simulink model "Controller_Sim"  (R2016a)
settings: Solver=ode1  SolverMode=MultiTasking  StartTime=0.0  StopTime=10  FixedStep=0.0005  RelTol=1e-3
StopFcn:
  | structifySimData
  | ConstructLog_Sim
values from neighbouring files (symbols this model uses):
  ControlParams = input.ControlParams    [Controller.m]    (also in Controller_Yukai.m)
  ControlState = input.ControlState    [Controller.m]    (also in Controller_Yukai.m)
undefined symbols (not defined in the file or in its folder): DiscIntNeverNeededParam, EnablePerturb, EnableStictionModel, FootPoints, gd, get, GroundModel, leg_length, LegHipTorqueLimit, LibWalkingDDA, pL1, pL2, pR1, pR2, ps3Axes, ps3Buttons, ps3Pov, RoughTerrain1, spring_k, spring_zeta, torso_com_offset, Ts, xinit, xLine, yLine, Z
libraries: simulink x5, Friction_Compensator_Lib x2, robotlib x2, vrlib x1
(part 1 of 2)
settings Model: ParamWorkspaceSource=ReferencedWorkspace  TunableVars=AllowDoubleSupport,Alpha0Frottement,Alpha2Frottement,BoomParams,ControlParams,ControlState,ControllerModeInit,EnablePerturb,EnableTransition,EnergyControlGain,EnergyControlPhi0,GaitLibrary,HipPushMag,KASaturationEarly,KASaturationMax,KASaturationS1,KASaturationS2,KASpringOffsets,KContact,KZeroYaw,K_sha,K_sla,Ksqrt,KsqrtVert,LambdaContact,LegHipTorqueLimit,MinDeltaThetaTransition,ProjectTo2D,RunMode,SWAP_DELAY,StanceLegInit,TMaxUpdate,TPosing,TorsoBackAngle,TorsoBackOnStep,TransitionOutputParams,UseKASaturation,UsePosingControl,VBLAOptions,WalkingOutputParams,balanceParams,enable_dx_tgt,enable_dy_tgt,enable_sideStep,enable_yawControl,epsilon,ff_params,foot_adjust_params,foot_geometry,foot_points,ground_coefficient_of_friction,ground_height_data,h_alpha_nom,h_alpha_transition,hd_posing,isTest_constantHips,isTest_doubleSupport,isTest_hipTracking,isTest_holdInAir,isTest_stopAndGo,k_precomp,kd,kd_2dof,kd_hip,kd_pitch,kd_roll,kd_sha,kd_sla,kd_st_leg,kd_stanceHip,kd_stanceKnee,kd_stanceLeg,kd_sw_leg,kd_swingHip,kd_swingKnee,kd_swingLeg,kd_torso,ki_sha,ki_sla,kp,kp_2dof,kp_hip,kp_pitch,kp_roll,kp_sha,kp_sla,kp_st_leg,kp_stanceHip,kp_stanceKnee,kp_stanceLeg,kp_sw_leg,kp_swingHip,kp_swingKnee,kp_swingLeg,kp_torso,kp_yaw,lat_bias,lateralParams,optimal_sat_weights,pBInitial,ps3Axes,ps3Buttons,ps3Pov,springDeflectionImpactThreshold,spring_k,spring_zeta,stepTime,step_params,swap_params,swingHipAdjustmentGain,swingLegAdjustmentGain,tStepInitial,theta_limits_nom,theta_limits_transition,thres_hi,thres_lo,transitionParams,uHipGravity,u_ff,use2DOFHipControl,useConstantDecoupling,useOptimalSaturation,use_state_estimator,viscous_friction_yaw_constant,w_torso_lat,xinit  TunableVarsStorageClass=Auto,Auto,Auto,Auto,Auto,Auto,Auto,Auto,Auto,Auto,Auto,Auto,Auto,Auto,Auto,Auto,Auto,Auto,Auto,Auto,Auto,Auto,Auto,Auto,Auto,Auto,Auto,Auto,Auto,Auto,Auto,Auto,Auto,Auto,Auto,Auto,Auto,Auto,Auto,Auto,Auto,Auto,Auto,Auto,Auto,Auto,Auto,Auto,Auto,Auto,Auto,Auto,Auto,Auto,Auto,Auto,Auto,Auto,Auto,Auto,Auto,Auto,Auto,Auto,Auto,Auto,Auto,Auto,Auto,Auto,Auto,Auto,Auto,Auto,Auto,Auto,Auto,Auto,Auto,Auto,Auto,Auto,Auto,Auto,Auto,Auto,Auto,Auto,Auto,Auto,Auto,Auto,Auto,Auto,Auto,Auto,Auto,Auto,Auto,Auto,Auto,Auto,Auto,Auto,Auto,Auto,Auto,Auto,Auto,Auto,Auto,Auto,Auto,Auto,Auto,Auto,Auto,Auto,Auto,Auto,Auto,Auto,Auto,Auto,Auto,Auto  TunableVarsTypeQualifier=,,,,,,,,,,,,,,,,,,,,,,,,,,,,,,,,,,,,,,,,,,,,,,,,,,,,,,,,,,,,,,,,,,,,,,,,,,,,,,,,,,,,,,,,,,,,,,,,,,,,,,,,,,,,,,,,,,,,,,,,,,,,,  Creator=kevinsg  LastModifiedBy=gyk
settings SolverCC: AlgebraicLoopSolver=LineSearch
settings DataIOCC: LimitDataPoints=on  SaveFormat=Array
settings OptimizationCC: BlockReduction=off  BooleanDataType=off
settings DebuggingCC: SaveWithParameterizedLinksMsg=none  SignalResolutionControl=TryResolveAllWithWarning  AllowSymbolicDim=off
settings HardwareCC: ProdBitPerPointer=32  ProdLargestAtomicFloat=None  ProdIntDivRoundTo=Undefined  ProdEndianess=Unspecified  ProdWordSize=32  ProdHWDeviceType=32-bit Generic  TargetBitPerPointer=64  TargetLongLongMode=on  TargetIntDivRoundTo=Zero  TargetEndianess=LittleEndian  TargetWordSize=64  TargetHWDeviceType=MATLAB Host  ProdEqTarget=off
settings ModelReferenceCC: PropagateSignalLabelsOutOfModel=off
settings ConfigComp: CovModelRefEnable=Off  CovSFcnEnable=off

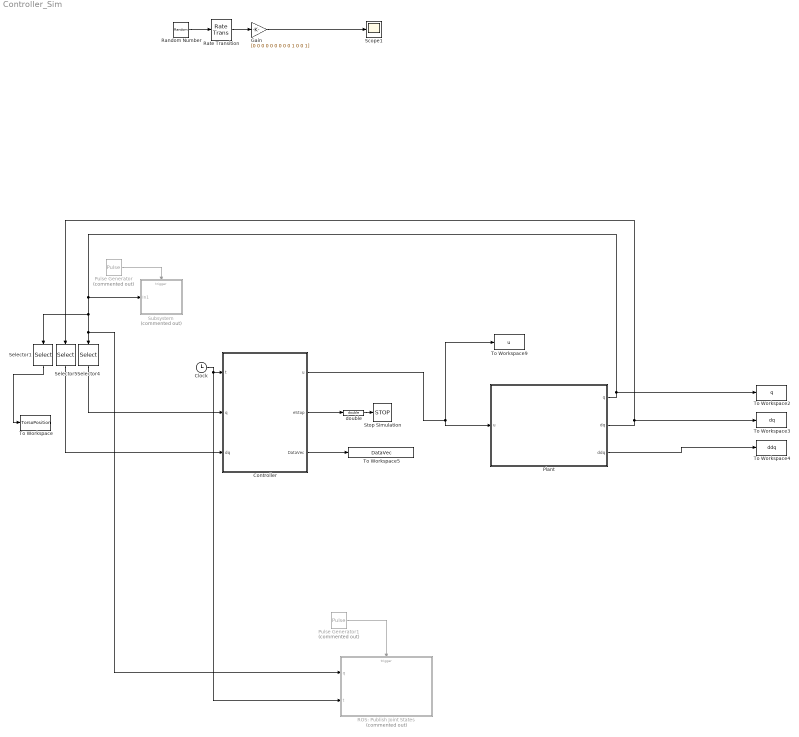
== system Controller_Sim ==
  Clock : Clock
  Controller : Subsystem  AncestorBlock=LibWalkingDDA/RoughTerrain1
  Gain : Gain  Gain=[0 0 0 0 0 0 0 0 0 1 0 0 1]
  Plant : Subsystem
  Pulse Generator : DiscretePulseGenerator  Commented=on  PulseType=Time based  Period=.01  PulseWidth=5
  Pulse Generator1 : DiscretePulseGenerator  Commented=on  PulseType=Time based  Period=.01  PulseWidth=5
  ROS: Publish Joint States : Subsystem  Commented=on
  Random Number : RandomNumber  Variance=Ts*300  SampleTime=Ts*100
  Rate Transition : RateTransition  OutPortSampleTime=Ts
  Scope1 : Scope
  Selector1 : Selector  InputPortWidth=16  IndexOptions=Index vector (dialog)  Indices=[1,2,3,4,5,6]  OutputSizes=1
  Selector4 : Selector  InputPortWidth=16  IndexOptions=Index vector (dialog)  Indices=[4,5,6,7,8,9,10,11,12,13,14,15,16]  OutputSizes=1
  Selector5 : Selector  InputPortWidth=16  IndexOptions=Index vector (dialog)  Indices=[4,5,6,7,8,9,10,11,12,13,14,15,16]  OutputSizes=1
  Stop Simulation : Stop
  Subsystem : Subsystem  Commented=on
  To Workspace : ToWorkspace  VariableName=TorsoPosition  SampleTime=-1
      settings: Save2DSignal=2-D array (concatenate along first dimension)
  To Workspace2 : ToWorkspace  VariableName=q  SampleTime=-1
  To Workspace3 : ToWorkspace  VariableName=dq  SampleTime=-1
  To Workspace4 : ToWorkspace  VariableName=ddq  SampleTime=-1
  To Workspace5 : ToWorkspace  VariableName=DataVec  SampleTime=-1
  To Workspace9 : ToWorkspace  VariableName=u  SampleTime=-1
  double : DataTypeConversion  OutDataTypeStr=double
  wires:
  double/1 -> Stop Simulation/1
  Plant/3(ddq) -> To Workspace4/1
  Random Number/1 -> Rate Transition/1
  Rate Transition/1 -> Gain/1
  Gain/1 -> Scope1/1
  Selector4/1 -> Controller/2(q)
  Selector5/1 -> Controller/3(dq)
  Controller/3(DataVec) -> To Workspace5/1
  Controller/2(eStop) -> double/1
  Controller/1(u) -> To Workspace9/1, Plant/1(u)
  Plant/2(dq) -> To Workspace3/1, Selector5/1
  Pulse Generator/1 -> Subsystem/Trigger
  Clock/1 -> Controller/1(t), ROS: Publish Joint States/2(t)
  Plant/1(q) -> To Workspace2/1, Subsystem/1(In1), Selector1/1, ROS: Publish Joint States/1(q), Selector4/1
  Pulse Generator1/1 -> ROS: Publish Joint States/Trigger
  Selector1/1 -> To Workspace/1

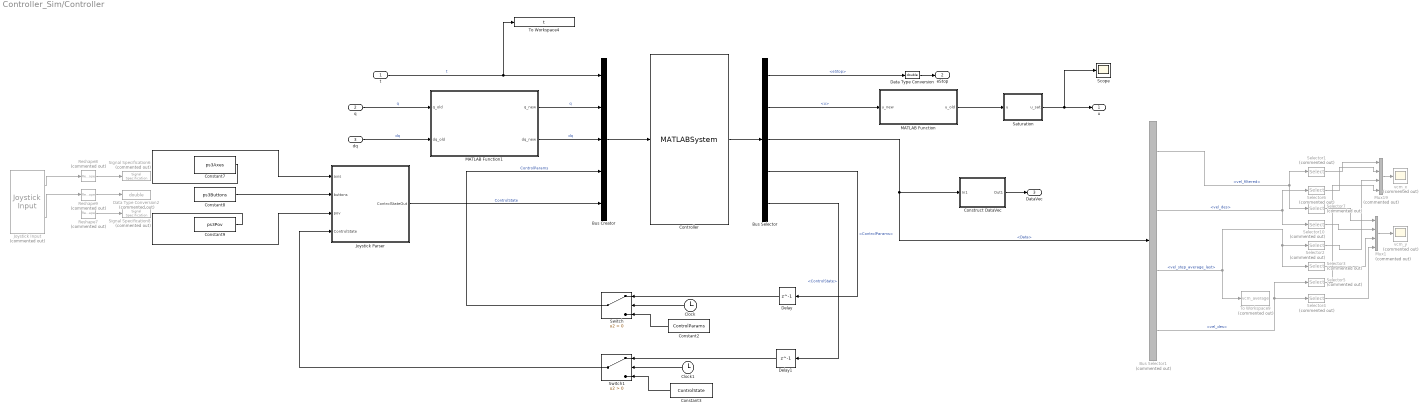
== system Controller_Sim/Controller ==
  t : Inport
  q : Inport  Port=2
  dq : Inport  Port=3
  Bus Creator : BusCreator  Inputs='t','q','dq','ControlParams','ControlState'  OutDataTypeStr=Bus: Input_bus
  Bus Selector : BusSelector  OutputSignals=eStop,u,Data,ControlParams,ControlState
  Bus Selector1 : BusSelector  Commented=on  OutputSignals=vel_filtered,vel_des,vel_step_average_last,vel_des
  Clock : Clock
  Clock1 : Clock
  Constant2 : Constant  Value=ControlParams  OutDataTypeStr=Bus: ControlParams_bus
  Constant3 : Constant  Value=ControlState  OutDataTypeStr=Bus: ControlState_bus
  Constant7 : Constant  Value=ps3Axes
  Constant8 : Constant  Value=ps3Buttons
  Constant9 : Constant  Value=ps3Pov
  Construct DataVec : Subsystem
  Controller : MATLABSystem  System=Controller  isSim=true  OutputBusName=Output_bus  SimulateUsing=Code generation
      mask Type: Controller
      mask Display:
      | disp('Controller');
      | port_label('input',1,'input');
      | port_label('output',1,'output');
  Data Type Conversion : DataTypeConversion  OutDataTypeStr=double
  Data Type Conversion2 : DataTypeConversion  Commented=on  OutDataTypeStr=double
  Delay : Delay  DelayLength=1  InitialCondition=0  InputProcessing=Inherited
  Delay1 : Delay  DelayLength=1  InitialCondition=0  InputProcessing=Inherited
  Joystick Input : vrlib/Joystick Input  Commented=on  joyid=1  adjustports=on  forcefeed=off
  Joystick Parser : Subsystem
  MATLAB Function : MATLAB Function  TreatAsAtomicUnit=on
  MATLAB Function1 : MATLAB Function  TreatAsAtomicUnit=on
  Mux1 : Mux  Commented=on
  Mux19 : Mux  Commented=on
  Reshape7 : Reshape  Commented=on  OutputDimensionality=Row vector (2-D)
  Reshape8 : Reshape  Commented=on  OutputDimensionality=Row vector (2-D)
  Reshape9 : Reshape  Commented=on  OutputDimensionality=Row vector (2-D)
  Saturation : Subsystem
  Scope : Scope
  Selector{1..2,5..6} (4 alike) : Selector  Commented=on  InputPortWidth=3  IndexOptions=Index vector (dialog)  Indices=[1]  OutputSizes=1
  Selector{3..4,7,10} (4 alike) : Selector  Commented=on  InputPortWidth=3  IndexOptions=Index vector (dialog)  Indices=[2]  OutputSizes=1
  Signal Specification6 : SignalSpecification  Commented=on  OutDataTypeStr=double  Dimensions=5
  Signal Specification8 : SignalSpecification  Commented=on  OutDataTypeStr=double
  Switch : Switch  Criteria=u2 > Threshold
  Switch1 : Switch  Criteria=u2 > Threshold
  To Workspace4 : ToWorkspace  VariableName=t  SampleTime=-1
  To Workspace9 : ToWorkspace  Commented=on  VariableName=vcm_average  SampleTime=-1
  vcm_x : Scope  Commented=on
  vcm_y : Scope  Commented=on
  u : Outport  OutDataTypeStr=double
  eStop : Outport  Port=2  OutDataTypeStr=double
  DataVec : Outport  Port=3
  wires:
  Joystick Parser/1(ControlStateOut) -> Bus Creator/5  "ControlState"
  Switch/1 -> Bus Creator/4  "ControlParams"
  dq/1 -> MATLAB Function1/2(dq_old)  "dq"
  Bus Selector/1 -> Data Type Conversion/1  "<eStop>"
  Data Type Conversion/1 -> eStop/1
  Saturation/1(u_sat) -> Scope/1, u/1
  t/1 -> To Workspace4/1, Bus Creator/1  "t"
  Bus Creator/1 -> Controller/1
  Controller/1 -> Bus Selector/1
  Bus Selector/3 -> Bus Selector1/1, Construct DataVec/1(In1)  "<Data>"
  Bus Selector/4 -> Delay/1  "<ControlParams>"
  Bus Selector/5 -> Delay1/1  "<ControlState>"
  Delay/1 -> Switch/1
  Delay1/1 -> Switch1/1
  Clock/1 -> Switch/2
  Constant2/1 -> Switch/3
  Clock1/1 -> Switch1/2
  Constant3/1 -> Switch1/3
  Switch1/1 -> Joystick Parser/4(ControlState)
  Mux19/1 -> vcm_x/1
  Bus Selector1/1 -> Selector1/1, Selector7/1  "<vel_filtered>"
  Bus Selector1/2 -> Selector6/1, Selector10/1  "<vel_des>"
  Selector6/1 -> Mux19/2
  Selector1/1 -> Mux19/1
  Mux1/1 -> vcm_y/1
  Selector10/1 -> Mux1/2
  Selector7/1 -> Mux1/1
  Bus Selector1/3 -> Selector3/1, Selector2/1, To Workspace9/1  "<vel_step_average_last>"
  Selector2/1 -> Mux19/3
  Selector3/1 -> Mux1/3
  Joystick Input/2 -> Reshape9/1
  Reshape8/1 -> Signal Specification6/1
  Joystick Input/1 -> Reshape8/1
  Reshape7/1 -> Signal Specification8/1
  ? -> Reshape7/1
  Reshape9/1 -> Data Type Conversion2/1
  Construct DataVec/1(Out1) -> DataVec/1
  Constant7/1 -> Joystick Parser/1(axis)
  Constant8/1 -> Joystick Parser/2(buttons)
  Constant9/1 -> Joystick Parser/3(pov)
  Selector4/1 -> Mux1/4
  Bus Selector1/4 -> Selector5/1, Selector4/1  "<vel_des>"
  Selector5/1 -> Mux19/4
  q/1 -> MATLAB Function1/1(q_old)  "q"
  MATLAB Function1/1(q_new) -> Bus Creator/2  "q"
  MATLAB Function/1(u_old) -> Saturation/1(u)
  Bus Selector/2 -> MATLAB Function/1(u_new)  "<u>"
  MATLAB Function1/2(dq_new) -> Bus Creator/3  "dq"

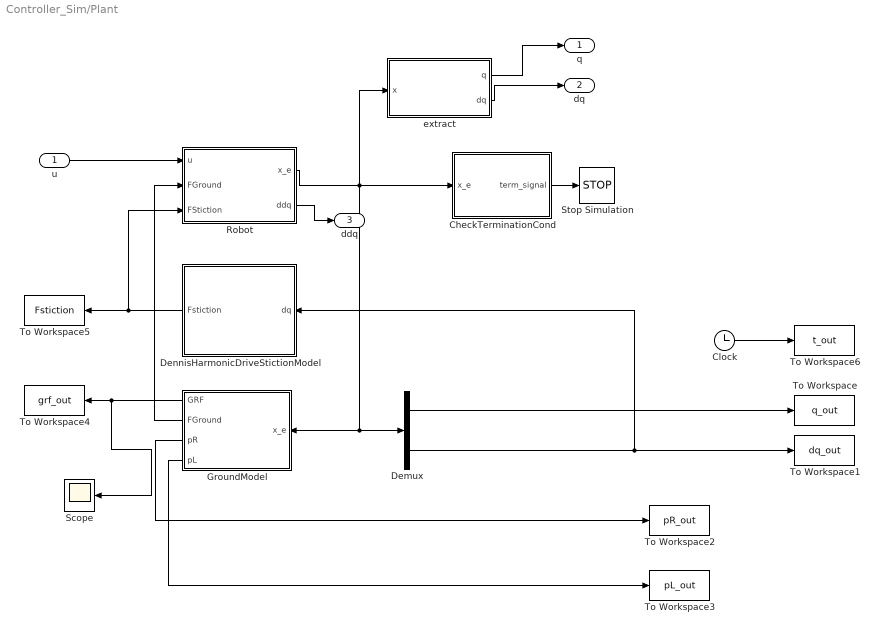
== system Controller_Sim/Plant ==
  u : Inport
  CheckTerminationCond : Subsystem
  Clock : Clock
  Demux : Demux  Outputs=[16 16]
  DennisHarmonicDriveStictionModel : Subsystem
  GroundModel : Subsystem
  Robot : Subsystem
  Scope : Scope
  Stop Simulation : Stop
  To Workspace : ToWorkspace  VariableName=q_out  SampleTime=-1
  To Workspace1 : ToWorkspace  VariableName=dq_out  SampleTime=-1
  To Workspace2 : ToWorkspace  VariableName=pR_out  SampleTime=-1
  To Workspace3 : ToWorkspace  VariableName=pL_out  SampleTime=-1
  To Workspace4 : ToWorkspace  VariableName=grf_out  SampleTime=-1
  To Workspace5 : ToWorkspace  VariableName=Fstiction  SampleTime=-1
  To Workspace6 : ToWorkspace  VariableName=t_out  SampleTime=-1
  extract : MATLAB Function  TreatAsAtomicUnit=on
  q : Outport
  dq : Outport  Port=2
  ddq : Outport  Port=3
  wires:
  Robot/1(x_e) -> extract/1(x), GroundModel/1(x_e), Demux/1, CheckTerminationCond/1(x_e)
  GroundModel/2(FGround) -> Robot/2(FGround)
  Demux/2 -> DennisHarmonicDriveStictionModel/1(dq), To Workspace1/1
  Demux/1 -> To Workspace/1
  CheckTerminationCond/1(term_signal) -> Stop Simulation/1
  u/1 -> Robot/1(u)
  extract/1(q) -> q/1
  GroundModel/1(GRF) -> Scope/1, To Workspace4/1
  GroundModel/3(pR) -> To Workspace2/1
  GroundModel/4(pL) -> To Workspace3/1
  DennisHarmonicDriveStictionModel/1(Fstiction) -> To Workspace5/1, Robot/3(FStiction)
  extract/2(dq) -> dq/1
  Clock/1 -> To Workspace6/1
  Robot/2(ddq) -> ddq/1

== system Controller_Sim/ROS: Publish Joint States ==
  q : Inport
  t : Inport  Port=2
  Trigger : TriggerPort  VariantControl=Variant  PortDimensions=1
  Blank Message1 : robotlib/Blank Message  SourceLibraryInfo=This block requires Robotics System Toolbox  messageType=trajectory_msgs/JointTrajectory  SampleTime=inf
  Constant7 : Constant  Value=Ts
  MATLAB Function - Assign : MATLAB Function  TreatAsAtomicUnit=on
  Publish : robotlib/Publish  SourceLibraryInfo=This block requires Robotics System Toolbox  topicSource=Specify your own  topic=/set_joint_trajectory  messageType=trajectory_msgs/JointTrajectory  messageQueueLength=1
  wires:
  MATLAB Function - Assign/1(msg) -> Publish/1
  Blank Message1/1 -> MATLAB Function - Assign/1(blankMessage)
  t/1 -> MATLAB Function - Assign/2(t)
  q/1 -> MATLAB Function - Assign/3(q)
  Constant7/1 -> MATLAB Function - Assign/4(Ts)

== system Controller_Sim/Subsystem ==
  In1 : Inport
  Trigger : TriggerPort  VariantControl=Variant  PortDimensions=1
  MATLAB Function : MATLAB Function  TreatAsAtomicUnit=on
  torso_com_offset : Constant  Value=torso_com_offset
  torso_com_offset1 : Constant  Value=leg_length
  wires:
  In1/1 -> MATLAB Function/1(q)
  torso_com_offset1/1 -> MATLAB Function/2(leg_length)
  torso_com_offset/1 -> MATLAB Function/3(torso_com_offset)

== system Controller_Sim/Controller/Construct DataVec ==
  In1 : Inport
  DataBusSelector : BusSelector  OutputSignals=q,dq,u,y,dy,s,cs,hd,dhd,h0,dh0,pitch_tune,roll_tune,pitch_tune_fil,roll_tune_fil
  DataVectorize : Concatenate  NumInputs=15
  Out1 : Outport
  wires:
  In1/1 -> DataBusSelector/1
  DataVectorize/1 -> Out1/1
  DataBusSelector/1 -> DataVectorize/1  "<q>"
  DataBusSelector/2 -> DataVectorize/2  "<dq>"
  DataBusSelector/3 -> DataVectorize/3  "<u>"
  DataBusSelector/4 -> DataVectorize/4  "<y>"
  DataBusSelector/5 -> DataVectorize/5  "<dy>"
  DataBusSelector/6 -> DataVectorize/6  "<s>"
  DataBusSelector/7 -> DataVectorize/7  "<cs>"
  DataBusSelector/8 -> DataVectorize/8  "<hd>"
  DataBusSelector/9 -> DataVectorize/9  "<dhd>"
  DataBusSelector/10 -> DataVectorize/10  "<h0>"
  DataBusSelector/11 -> DataVectorize/11  "<dh0>"
  DataBusSelector/12 -> DataVectorize/12  "<pitch_tune>"
  DataBusSelector/13 -> DataVectorize/13  "<roll_tune>"
  DataBusSelector/14 -> DataVectorize/14  "<pitch_tune_fil>"
  DataBusSelector/15 -> DataVectorize/15  "<roll_tune_fil>"

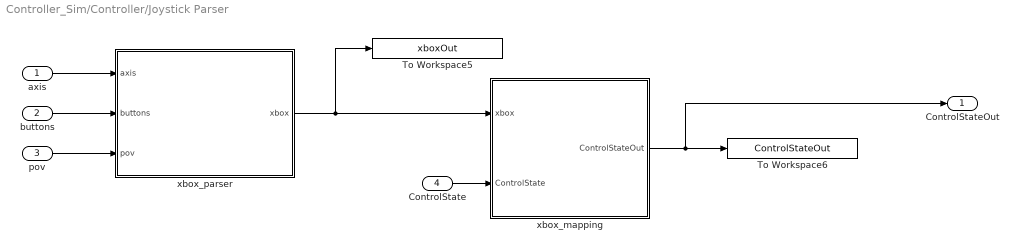
== system Controller_Sim/Controller/Joystick Parser ==
  axis : Inport
  buttons : Inport  Port=2
  pov : Inport  Port=3
  ControlState : Inport  Port=4  OutDataTypeStr=Bus: ControlState_bus
  To Workspace5 : ToWorkspace  VariableName=xboxOut  SaveFormat=Timeseries  SampleTime=-1
  To Workspace6 : ToWorkspace  VariableName=ControlStateOut  SaveFormat=Timeseries  SampleTime=-1
  xbox_mapping : Subsystem
  xbox_parser : MATLAB Function  TreatAsAtomicUnit=on
  ControlStateOut : Outport  OutDataTypeStr=Bus: ControlState_bus
  wires:
  xbox_parser/1(xbox) -> To Workspace5/1, xbox_mapping/1(xbox)
  xbox_mapping/1(ControlStateOut) -> To Workspace6/1, ControlStateOut/1
  axis/1 -> xbox_parser/1(axis)
  buttons/1 -> xbox_parser/2(buttons)
  pov/1 -> xbox_parser/3(pov)
  ControlState/1 -> xbox_mapping/2(ControlState)

== system Controller_Sim/Controller/Saturation ==
  u : Inport
  Data Type Conversion1 : DataTypeConversion  OutDataTypeStr=double
  Gain : Gain  Gain=-1
  Gain1 : Gain  Gain=[1 0; 1 0; 0 1; 1 0; 1 0; 0 1]  Multiplication=Matrix(K*u)
  LegHipTorqueSat : Constant  Value=LegHipTorqueLimit
  Saturation Dynamic : simulink/Discontinuities/Saturation Dynamic  OutMin=[]  OutMax=[]  OutDataTypeStr=Inherit: Same as second input  OutDataType=fixdt(1, 16)  OutScaling=2^-10  DoSatur=off
  u_sat : Outport  OutDataTypeStr=double
  wires:
  Saturation Dynamic/1 -> Data Type Conversion1/1
  Data Type Conversion1/1 -> u_sat/1  "torque_sat"
  LegHipTorqueSat/1 -> Gain1/1
  Gain1/1 -> Saturation Dynamic/1, Gain/1
  Gain/1 -> Saturation Dynamic/3
  u/1 -> Saturation Dynamic/2

== system Controller_Sim/Plant/CheckTerminationCond ==
  x_e : Inport
  MATLAB Function : MATLAB Function  TreatAsAtomicUnit=on
  torso_com_offset : Constant  Value=torso_com_offset
  torso_com_offset1 : Constant  Value=leg_length
  term_signal : Outport
  wires:
  x_e/1 -> MATLAB Function/1(x_e)
  MATLAB Function/1(terminate_signal) -> term_signal/1
  torso_com_offset1/1 -> MATLAB Function/2(leg_length)
  torso_com_offset/1 -> MATLAB Function/3(torso_com_offset)

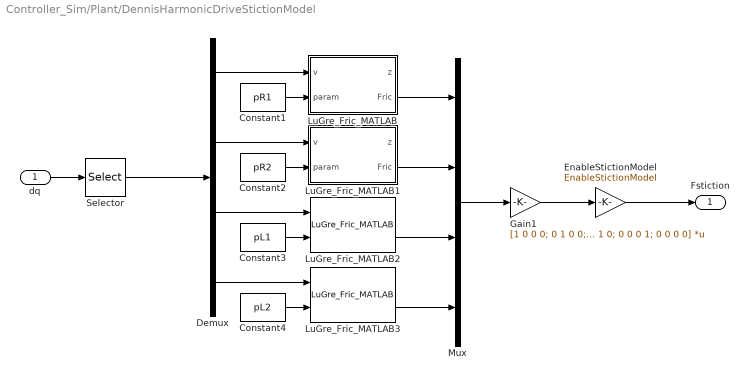
== system Controller_Sim/Plant/DennisHarmonicDriveStictionModel ==
  dq : Inport
  Constant1 : Constant  Value=pR1
  Constant2 : Constant  Value=pR2
  Constant3 : Constant  Value=pL1
  Constant4 : Constant  Value=pL2
  Demux : Demux
  EnableStictionModel : Gain  Gain=EnableStictionModel
  Gain1 : Gain  Gain=[1 0 0 0; 0 1 0 0; 0 0 0 0; 0 0 1 0; 0 0 0 1; 0 0 0 0]  Multiplication=Matrix(K*u)
  LuGre_Fric_MATLAB : Subsystem  AncestorBlock=Friction_Compensator_Lib/LuGre_Fric_MATLAB
  LuGre_Fric_MATLAB1 : Subsystem  AncestorBlock=Friction_Compensator_Lib/LuGre_Fric_MATLAB
  LuGre_Fric_MATLAB2 : Friction_Compensator_Lib/LuGre_Fric_MATLAB
  LuGre_Fric_MATLAB3 : Friction_Compensator_Lib/LuGre_Fric_MATLAB
  Mux : Mux
  Selector : Selector  InputPortWidth=16  IndexOptions=Index vector (dialog)  Indices=[11 12 14 15]  OutputSizes=1
  Fstiction : Outport
  wires:
  dq/1 -> Selector/1
  Selector/1 -> Demux/1
  EnableStictionModel/1 -> Fstiction/1
  Gain1/1 -> EnableStictionModel/1
  Constant1/1 -> LuGre_Fric_MATLAB/2(param)
  Constant2/1 -> LuGre_Fric_MATLAB1/2(param)
  Constant3/1 -> LuGre_Fric_MATLAB2/2
  Constant4/1 -> LuGre_Fric_MATLAB3/2
  Demux/4 -> LuGre_Fric_MATLAB3/1
  Demux/3 -> LuGre_Fric_MATLAB2/1
  Demux/2 -> LuGre_Fric_MATLAB1/1(v)
  Demux/1 -> LuGre_Fric_MATLAB/1(v)
  LuGre_Fric_MATLAB/2(Fric) -> Mux/1
  LuGre_Fric_MATLAB1/2(Fric) -> Mux/2
  LuGre_Fric_MATLAB2/2 -> Mux/3
  LuGre_Fric_MATLAB3/2 -> Mux/4
  Mux/1 -> Gain1/1

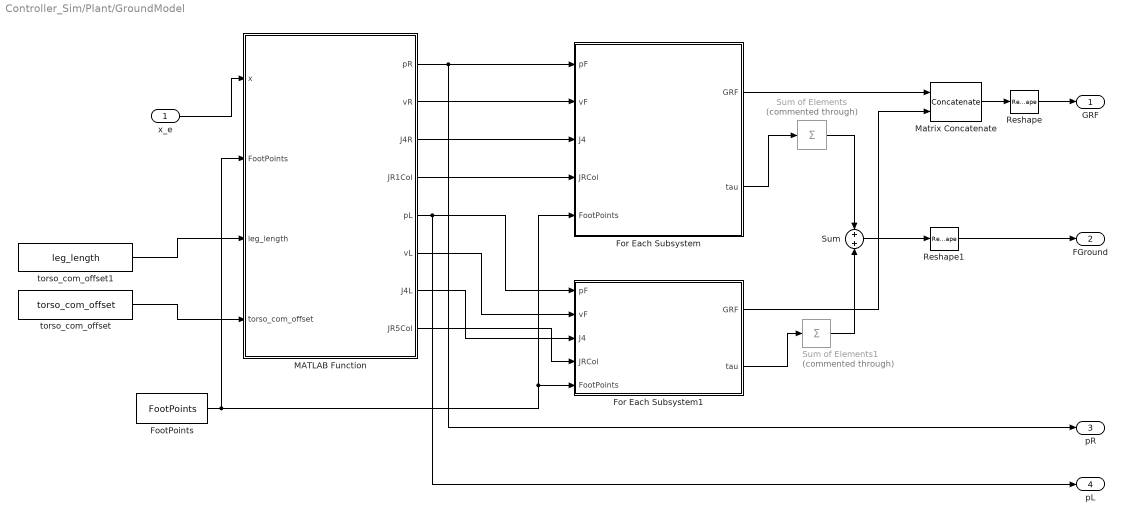
== system Controller_Sim/Plant/GroundModel ==
  x_e : Inport
  FootPoints : Constant  Value=FootPoints
  For Each Subsystem : Subsystem  TreatAsAtomicUnit=on
  For Each Subsystem1 : Subsystem  TreatAsAtomicUnit=on
  MATLAB Function : MATLAB Function  TreatAsAtomicUnit=on
  Matrix Concatenate : Concatenate  Mode=Multidimensional array
  Reshape : Reshape
  Reshape1 : Reshape
  Sum : Sum  Inputs=+|+
  Sum of Elements : Sum  Commented=through  Inputs=+  CollapseMode=Specified dimension  CollapseDim=2
  Sum of Elements1 : Sum  Commented=through  Inputs=+  CollapseMode=Specified dimension  CollapseDim=2
  torso_com_offset : Constant  Value=torso_com_offset
  torso_com_offset1 : Constant  Value=leg_length
  GRF : Outport
  FGround : Outport  Port=2
  pR : Outport  Port=3
  pL : Outport  Port=4
  wires:
  x_e/1 -> MATLAB Function/1(x)
  MATLAB Function/1(pR) -> pR/1, For Each Subsystem/1(pF)
  For Each Subsystem/1(GRF) -> Matrix Concatenate/1
  Matrix Concatenate/1 -> Reshape/1
  For Each Subsystem1/1(GRF) -> Matrix Concatenate/2
  Reshape/1 -> GRF/1
  MATLAB Function/2(vR) -> For Each Subsystem/2(vF)
  MATLAB Function/3(J4R) -> For Each Subsystem/3(J4)
  MATLAB Function/4(JR1Col) -> For Each Subsystem/4(JRCol)
  MATLAB Function/5(pL) -> For Each Subsystem1/1(pF), pL/1
  MATLAB Function/6(vL) -> For Each Subsystem1/2(vF)
  MATLAB Function/7(J4L) -> For Each Subsystem1/3(J4)
  MATLAB Function/8(JR5Col) -> For Each Subsystem1/4(JRCol)
  FootPoints/1 -> MATLAB Function/2(FootPoints), For Each Subsystem/5(FootPoints), For Each Subsystem1/5(FootPoints)
  For Each Subsystem/2(tau) -> Sum of Elements/1
  For Each Subsystem1/2(tau) -> Sum of Elements1/1
  Sum of Elements/1 -> Sum/1
  Sum of Elements1/1 -> Sum/2
  Sum/1 -> Reshape1/1
  Reshape1/1 -> FGround/1
  torso_com_offset1/1 -> MATLAB Function/3(leg_length)
  torso_com_offset/1 -> MATLAB Function/4(torso_com_offset)

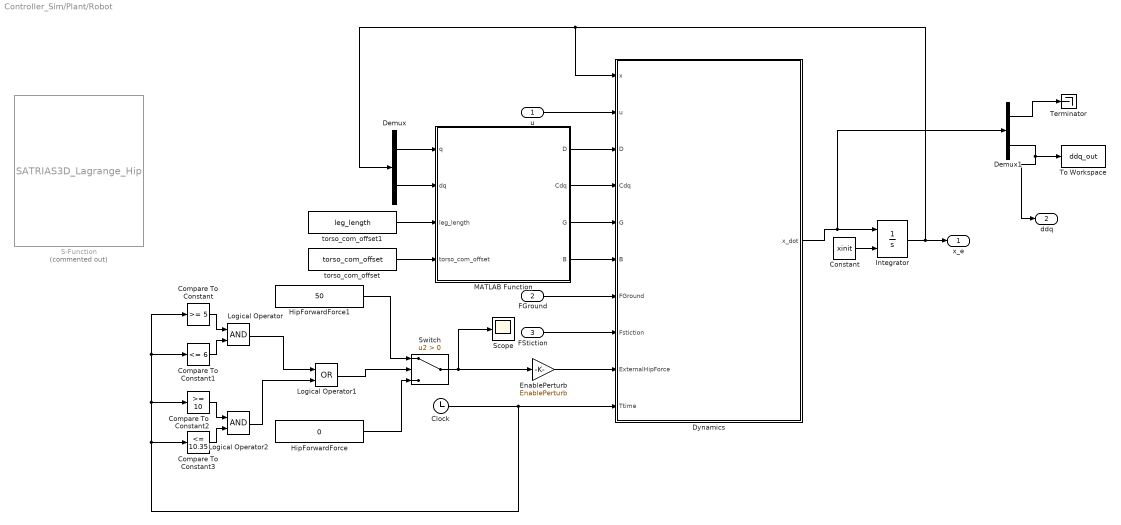
== system Controller_Sim/Plant/Robot ==
  u : Inport
  FGround : Inport  Port=2
  FStiction : Inport  Port=3
  Clock : Clock
  Compare To Constant : simulink/Logic and Bit Operations/Compare To Constant  relop=>=  const=5  OutDataTypeStr=boolean
  Compare To Constant1 : simulink/Logic and Bit Operations/Compare To Constant  relop=<=  const=6  OutDataTypeStr=boolean
  Compare To Constant2 : simulink/Logic and Bit Operations/Compare To Constant  relop=>=  const=10  OutDataTypeStr=boolean
  Compare To Constant3 : simulink/Logic and Bit Operations/Compare To Constant  relop=<=  const=10.35  OutDataTypeStr=boolean
  Constant : Constant  Value=xinit
  Demux : Demux  Outputs=[16 16]
  Demux1 : Demux  Outputs=[16 16]
  Dynamics : MATLAB Function  TreatAsAtomicUnit=on
  EnablePerturb : Gain  Gain=EnablePerturb
  HipForwardForce : Constant  Value=0
  HipForwardForce1 : Constant  Value=50  VectorParams1D=off
  Integrator : Integrator  InitialConditionSource=external  InitialCondition=str2num(get(gd.edit1,'string'))
  Logical Operator : Logic  AllPortsSameDT=off  OutDataTypeStr=boolean
  Logical Operator1 : Logic  Operator=OR  AllPortsSameDT=off  OutDataTypeStr=boolean
  Logical Operator2 : Logic  AllPortsSameDT=off  OutDataTypeStr=boolean
  MATLAB Function : MATLAB Function  TreatAsAtomicUnit=on
  S-Function : S-Function  Commented=on  FunctionName=SATRIAS3D_Lagrange_Hip  SFunctionModules='ATRIAS3D_D_Hip ATRIAS3D_Cdq_Hip ATRIAS3D_G_Hip ATRIAS3D_B_Hip'  SFunctionDeploymentMode=off  EnableBusSupport=off
      mask Display:
      | disp('ATRIAS3D_Lagrange_Hip')
      | port_label('input', 1, 'q')
      | port_label('input', 2, 'dq')
      | 
      | port_label('output', 1, 'D')
      | port_label('output', 2, 'Cdq')
      | port_label('output', 3, 'G')
      | port_label('output', 4, 'B')
  Scope : Scope
  Switch : Switch  Criteria=u2 > Threshold
  Terminator : Terminator
  To Workspace : ToWorkspace  VariableName=ddq_out  SampleTime=-1
  torso_com_offset : Constant  Value=torso_com_offset
  torso_com_offset1 : Constant  Value=leg_length
  x_e : Outport
  ddq : Outport  Port=2
  wires:
  FGround/1 -> Dynamics/7(FGround)
  u/1 -> Dynamics/2(u)
  Constant/1 -> Integrator/2
  Dynamics/1(x_dot) -> Demux1/1, Integrator/1
  Integrator/1 -> Dynamics/1(x), Demux/1, x_e/1
  HipForwardForce/1 -> Switch/3
  Clock/1 -> Compare To Constant3/1, Compare To Constant1/1, Compare To Constant/1, Compare To Constant2/1, Dynamics/10(Ttime)
  FStiction/1 -> Dynamics/8(Fstiction)
  HipForwardForce1/1 -> Switch/1
  Compare To Constant1/1 -> Logical Operator/2
  Compare To Constant/1 -> Logical Operator/1
  Logical Operator/1 -> Logical Operator1/1
  Switch/1 -> Scope/1, EnablePerturb/1
  EnablePerturb/1 -> Dynamics/9(ExternalHipForce)
  Demux1/2 -> ddq/1, To Workspace/1
  Demux1/1 -> Terminator/1
  Demux/1 -> MATLAB Function/1(q)
  Demux/2 -> MATLAB Function/2(dq)
  MATLAB Function/1(D) -> Dynamics/3(D)
  MATLAB Function/2(Cdq) -> Dynamics/4(Cdq)
  MATLAB Function/3(G) -> Dynamics/5(G)
  MATLAB Function/4(B) -> Dynamics/6(B)
  torso_com_offset/1 -> MATLAB Function/4(torso_com_offset)
  torso_com_offset1/1 -> MATLAB Function/3(leg_length)
  Logical Operator1/1 -> Switch/2
  Compare To Constant3/1 -> Logical Operator2/2
  Compare To Constant2/1 -> Logical Operator2/1
  Logical Operator2/1 -> Logical Operator1/2

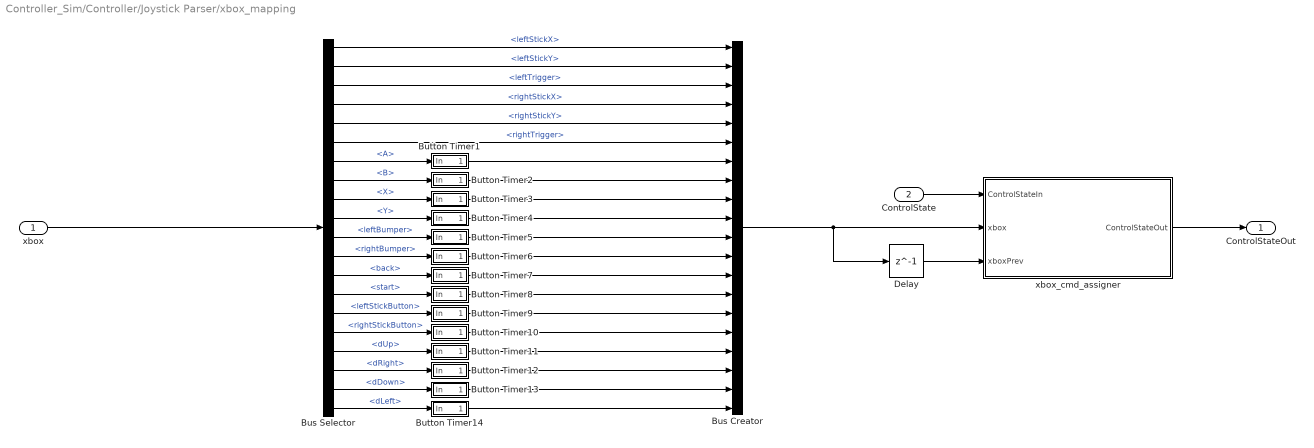
== system Controller_Sim/Controller/Joystick Parser/xbox_mapping ==
  xbox : Inport
  ControlState : Inport  Port=2  OutDataTypeStr=Bus: ControlState_bus
  Bus Creator : BusCreator  Inputs=20  OutDataTypeStr=Bus: xbox_bus  NonVirtualBus=on
  Bus Selector : BusSelector  OutputSignals=leftStickX,leftStickY,leftTrigger,rightStickX,rightStickY,rightTrigger,A,B,X,Y,leftBumper,rightBumper,back,start,leftStickButton,rightStickButton,dUp,dRight,dDown,dLeft
  Button Timer1 : Subsystem
  Button Timer10 : Subsystem
  Button Timer11 : Subsystem
  Button Timer12 : Subsystem
  Button Timer13 : Subsystem
  Button Timer14 : Subsystem
  Button Timer2 : Subsystem
  Button Timer3 : Subsystem
  Button Timer4 : Subsystem
  Button Timer5 : Subsystem
  Button Timer6 : Subsystem
  Button Timer7 : Subsystem
  Button Timer8 : Subsystem
  Button Timer9 : Subsystem
  Delay : Delay  DelayLength=1  InitialCondition=0
  xbox_cmd_assigner : MATLAB Function  TreatAsAtomicUnit=on
  ControlStateOut : Outport  OutDataTypeStr=Bus: ControlState_bus
  wires:
  Bus Selector/12 -> Button Timer6/1(In)  "<rightBumper>"
  Bus Selector/4 -> Bus Creator/4  "<rightStickX>"
  Bus Selector/3 -> Bus Creator/3  "<leftTrigger>"
  Bus Selector/9 -> Button Timer3/1(In)  "<X>"
  Bus Selector/1 -> Bus Creator/1  "<leftStickX>"
  Bus Selector/5 -> Bus Creator/5  "<rightStickY>"
  Bus Selector/14 -> Button Timer8/1(In)  "<start>"
  Bus Selector/17 -> Button Timer11/1(In)  "<dUp>"
  Bus Selector/18 -> Button Timer12/1(In)  "<dRight>"
  Bus Selector/8 -> Button Timer2/1(In)  "<B>"
  Bus Selector/19 -> Button Timer13/1(In)  "<dDown>"
  Bus Selector/7 -> Button Timer1/1(In)  "<A>"
  Bus Selector/15 -> Button Timer9/1(In)  "<leftStickButton>"
  xbox/1 -> Bus Selector/1
  Bus Selector/6 -> Bus Creator/6  "<rightTrigger>"
  Bus Selector/20 -> Button Timer14/1(In)  "<dLeft>"
  Bus Selector/2 -> Bus Creator/2  "<leftStickY>"
  Bus Selector/10 -> Button Timer4/1(In)  "<Y>"
  Bus Selector/13 -> Button Timer7/1(In)  "<back>"
  Bus Selector/16 -> Button Timer10/1(In)  "<rightStickButton>"
  Bus Selector/11 -> Button Timer5/1(In)  "<leftBumper>"
  Button Timer2/1(Out) -> Bus Creator/8
  Button Timer4/1(Out) -> Bus Creator/10
  Button Timer5/1(Out) -> Bus Creator/11
  Button Timer6/1(Out) -> Bus Creator/12
  Button Timer7/1(Out) -> Bus Creator/13
  Button Timer8/1(Out) -> Bus Creator/14
  Button Timer9/1(Out) -> Bus Creator/15
  Button Timer10/1(Out) -> Bus Creator/16
  Button Timer11/1(Out) -> Bus Creator/17
  Button Timer12/1(Out) -> Bus Creator/18
  Button Timer13/1(Out) -> Bus Creator/19
  Button Timer14/1(Out) -> Bus Creator/20
  Bus Creator/1 -> Delay/1, xbox_cmd_assigner/2(xbox)
  ControlState/1 -> xbox_cmd_assigner/1(ControlStateIn)
  Button Timer1/1(Out) -> Bus Creator/7
  Button Timer3/1(Out) -> Bus Creator/9
  xbox_cmd_assigner/1(ControlStateOut) -> ControlStateOut/1
  Delay/1 -> xbox_cmd_assigner/3(xboxPrev)

== system Controller_Sim/Plant/DennisHarmonicDriveStictionModel/LuGre_Fric_MATLAB ==
  note: The input unit is rad-based. In the MATLAB function, it will convert to deg-based value
  v : Inport
  param : Inport  Port=2
  Discrete-Time Integrator : DiscreteIntegrator  InitialConditionSetting=State (most efficient)  SampleTime=-1  ICPrevOutput=DiscIntNeverNeededParam  ICPrevScaledInput=DiscIntNeverNeededParam
  MATLAB Function : MATLAB Function  TreatAsAtomicUnit=on
  z : Outport
  Fric : Outport  Port=2
  wires:
  MATLAB Function/2(dz) -> Discrete-Time Integrator/1
  Discrete-Time Integrator/1 -> MATLAB Function/3(z), z/1
  MATLAB Function/1(Fric) -> Fric/1
  v/1 -> MATLAB Function/1(vel)
  param/1 -> MATLAB Function/2(p)

== system Controller_Sim/Plant/DennisHarmonicDriveStictionModel/LuGre_Fric_MATLAB1 ==
  note: The input unit is rad-based. In the MATLAB function, it will convert to deg-based value
  v : Inport
  param : Inport  Port=2
  Discrete-Time Integrator : DiscreteIntegrator  InitialConditionSetting=State (most efficient)  SampleTime=-1  ICPrevOutput=DiscIntNeverNeededParam  ICPrevScaledInput=DiscIntNeverNeededParam
  MATLAB Function : MATLAB Function  TreatAsAtomicUnit=on
  z : Outport
  Fric : Outport  Port=2
  wires:
  MATLAB Function/2(dz) -> Discrete-Time Integrator/1
  Discrete-Time Integrator/1 -> MATLAB Function/3(z), z/1
  MATLAB Function/1(Fric) -> Fric/1
  v/1 -> MATLAB Function/1(vel)
  param/1 -> MATLAB Function/2(p)

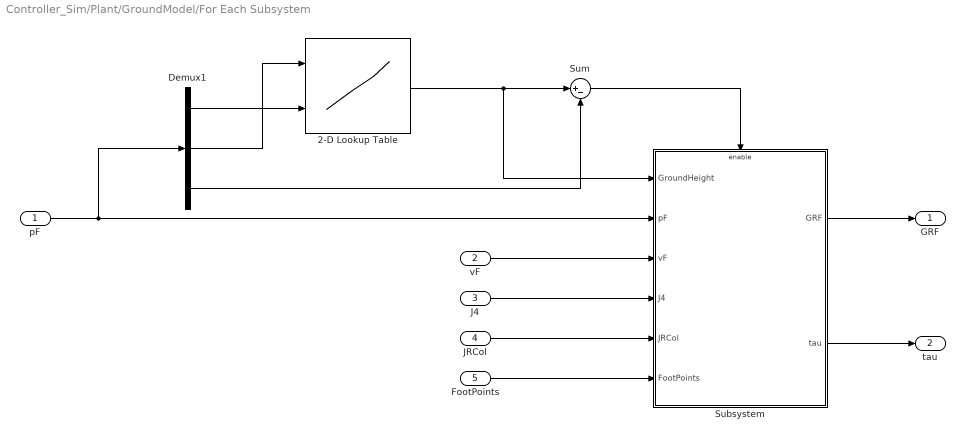
== system Controller_Sim/Plant/GroundModel/For Each Subsystem ==
  pF : Inport
  vF : Inport  Port=2
  J4 : Inport  Port=3
  JRCol : Inport  Port=4
  FootPoints : Inport  Port=5
  2-D Lookup Table : Lookup_n-D  BreakpointsForDimension1=xLine  BreakpointsForDimension2=yLine  Table=Z  InternalRulePriority=Speed  RndMeth=Simplest  InputSameDT=on
  Demux1 : Demux  Outputs=3
  Subsystem : Subsystem
  Sum : Sum  Inputs=|+-
  GRF : Outport
  tau : Outport  Port=2
  wires:
  vF/1 -> Subsystem/3(vF)
  J4/1 -> Subsystem/4(J4)
  JRCol/1 -> Subsystem/5(JRCol)
  FootPoints/1 -> Subsystem/6(FootPoints)
  Subsystem/2(tau) -> tau/1
  Sum/1 -> Subsystem/Enable
  Demux1/1 -> 2-D Lookup Table/2
  Demux1/2 -> 2-D Lookup Table/1
  pF/1 -> Subsystem/2(pF), Demux1/1
  2-D Lookup Table/1 -> Subsystem/1(GroundHeight), Sum/1
  Demux1/3 -> Sum/2
  Subsystem/1(GRF) -> GRF/1

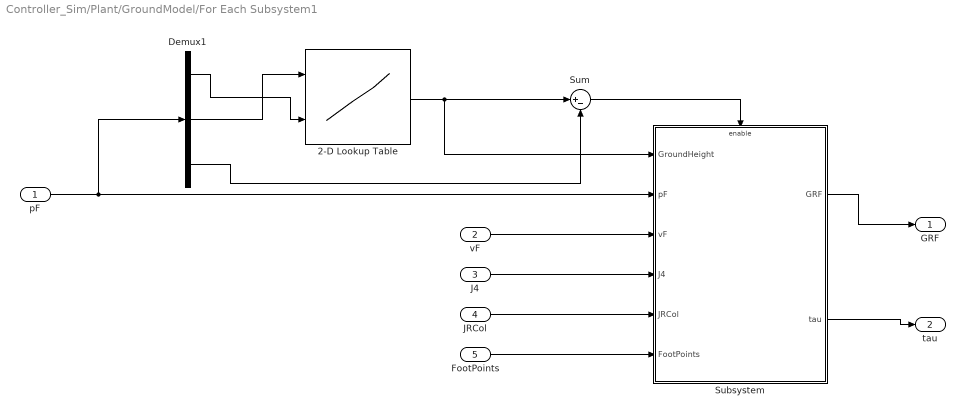
== system Controller_Sim/Plant/GroundModel/For Each Subsystem1 ==
  pF : Inport
  vF : Inport  Port=2
  J4 : Inport  Port=3
  JRCol : Inport  Port=4
  FootPoints : Inport  Port=5
  2-D Lookup Table : Lookup_n-D  BreakpointsForDimension1=xLine  BreakpointsForDimension2=yLine  Table=Z  InternalRulePriority=Speed  RndMeth=Simplest  InputSameDT=on
  Demux1 : Demux  Outputs=3
  Subsystem : Subsystem
  Sum : Sum  Inputs=|+-
  GRF : Outport
  tau : Outport  Port=2
  wires:
  Subsystem/1(GRF) -> GRF/1
  Demux1/3 -> Sum/2
  2-D Lookup Table/1 -> Sum/1, Subsystem/1(GroundHeight)
  pF/1 -> Demux1/1, Subsystem/2(pF)
  Demux1/2 -> 2-D Lookup Table/1
  Demux1/1 -> 2-D Lookup Table/2
  Sum/1 -> Subsystem/Enable
  Subsystem/2(tau) -> tau/1
  FootPoints/1 -> Subsystem/6(FootPoints)
  JRCol/1 -> Subsystem/5(JRCol)
  J4/1 -> Subsystem/4(J4)
  vF/1 -> Subsystem/3(vF)

== system Controller_Sim/Controller/Joystick Parser/xbox_mapping/Button Timer1 ==
  note: Button timer
      | Button needs to be pressed for 0.25 seconds to register
  In : Inport
  Clock : Clock
  Memory : Memory
  Sum : Sum  Inputs=|+-
  Switch : Switch  Criteria=u2 > Threshold
  Switch1 : Switch  Criteria=u2 > Threshold  Threshold=0.25
  off : Constant  Value=0
  on : Constant
  Out : Outport
  wires:
  off/1 -> Switch1/3
  Sum/1 -> Switch1/2
  Switch1/1 -> Out/1
  on/1 -> Switch1/1
  In/1 -> Switch/2
  Clock/1 -> Sum/1, Switch/3
  Memory/1 -> Switch/1
  Switch/1 -> Sum/2, Memory/1

== system Controller_Sim/Controller/Joystick Parser/xbox_mapping/Button Timer10 ==
  note: Button timer
      | Button needs to be pressed for 0.25 seconds to register
  In : Inport
  Clock : Clock
  Memory : Memory
  Sum : Sum  Inputs=|+-
  Switch : Switch  Criteria=u2 > Threshold
  Switch1 : Switch  Criteria=u2 > Threshold  Threshold=0.25
  off : Constant  Value=0
  on : Constant
  Out : Outport
  wires:
  off/1 -> Switch1/3
  Sum/1 -> Switch1/2
  Switch1/1 -> Out/1
  on/1 -> Switch1/1
  In/1 -> Switch/2
  Clock/1 -> Sum/1, Switch/3
  Memory/1 -> Switch/1
  Switch/1 -> Sum/2, Memory/1

== system Controller_Sim/Controller/Joystick Parser/xbox_mapping/Button Timer11 ==
  note: Button timer
      | Button needs to be pressed for 0.25 seconds to register
  In : Inport
  Clock : Clock
  Memory : Memory
  Sum : Sum  Inputs=|+-
  Switch : Switch  Criteria=u2 > Threshold
  Switch1 : Switch  Criteria=u2 > Threshold  Threshold=0.25
  off : Constant  Value=0
  on : Constant
  Out : Outport
  wires:
  off/1 -> Switch1/3
  Sum/1 -> Switch1/2
  Switch1/1 -> Out/1
  on/1 -> Switch1/1
  In/1 -> Switch/2
  Clock/1 -> Sum/1, Switch/3
  Memory/1 -> Switch/1
  Switch/1 -> Sum/2, Memory/1

== system Controller_Sim/Controller/Joystick Parser/xbox_mapping/Button Timer12 ==
  note: Button timer
      | Button needs to be pressed for 0.25 seconds to register
  In : Inport
  Clock : Clock
  Memory : Memory
  Sum : Sum  Inputs=|+-
  Switch : Switch  Criteria=u2 > Threshold
  Switch1 : Switch  Criteria=u2 > Threshold  Threshold=0.25
  off : Constant  Value=0
  on : Constant
  Out : Outport
  wires:
  off/1 -> Switch1/3
  Sum/1 -> Switch1/2
  Switch1/1 -> Out/1
  on/1 -> Switch1/1
  In/1 -> Switch/2
  Clock/1 -> Sum/1, Switch/3
  Memory/1 -> Switch/1
  Switch/1 -> Sum/2, Memory/1

== system Controller_Sim/Controller/Joystick Parser/xbox_mapping/Button Timer13 ==
  note: Button timer
      | Button needs to be pressed for 0.25 seconds to register
  In : Inport
  Clock : Clock
  Memory : Memory
  Sum : Sum  Inputs=|+-
  Switch : Switch  Criteria=u2 > Threshold
  Switch1 : Switch  Criteria=u2 > Threshold  Threshold=0.25
  off : Constant  Value=0
  on : Constant
  Out : Outport
  wires:
  off/1 -> Switch1/3
  Sum/1 -> Switch1/2
  Switch1/1 -> Out/1
  on/1 -> Switch1/1
  In/1 -> Switch/2
  Clock/1 -> Sum/1, Switch/3
  Memory/1 -> Switch/1
  Switch/1 -> Sum/2, Memory/1

== system Controller_Sim/Controller/Joystick Parser/xbox_mapping/Button Timer14 ==
  note: Button timer
      | Button needs to be pressed for 0.25 seconds to register
  In : Inport
  Clock : Clock
  Memory : Memory
  Sum : Sum  Inputs=|+-
  Switch : Switch  Criteria=u2 > Threshold
  Switch1 : Switch  Criteria=u2 > Threshold  Threshold=0.25
  off : Constant  Value=0
  on : Constant
  Out : Outport
  wires:
  off/1 -> Switch1/3
  Sum/1 -> Switch1/2
  Switch1/1 -> Out/1
  on/1 -> Switch1/1
  In/1 -> Switch/2
  Clock/1 -> Sum/1, Switch/3
  Memory/1 -> Switch/1
  Switch/1 -> Sum/2, Memory/1

== system Controller_Sim/Controller/Joystick Parser/xbox_mapping/Button Timer2 ==
  note: Button timer
      | Button needs to be pressed for 0.25 seconds to register
  In : Inport
  Clock : Clock
  Memory : Memory
  Sum : Sum  Inputs=|+-
  Switch : Switch  Criteria=u2 > Threshold
  Switch1 : Switch  Criteria=u2 > Threshold  Threshold=0.25
  off : Constant  Value=0
  on : Constant
  Out : Outport
  wires:
  off/1 -> Switch1/3
  Sum/1 -> Switch1/2
  Switch1/1 -> Out/1
  on/1 -> Switch1/1
  In/1 -> Switch/2
  Clock/1 -> Sum/1, Switch/3
  Memory/1 -> Switch/1
  Switch/1 -> Sum/2, Memory/1

== system Controller_Sim/Controller/Joystick Parser/xbox_mapping/Button Timer3 ==
  note: Button timer
      | Button needs to be pressed for 0.25 seconds to register
  In : Inport
  Clock : Clock
  Memory : Memory
  Sum : Sum  Inputs=|+-
  Switch : Switch  Criteria=u2 > Threshold
  Switch1 : Switch  Criteria=u2 > Threshold  Threshold=0.25
  off : Constant  Value=0
  on : Constant
  Out : Outport
  wires:
  off/1 -> Switch1/3
  Sum/1 -> Switch1/2
  Switch1/1 -> Out/1
  on/1 -> Switch1/1
  In/1 -> Switch/2
  Clock/1 -> Sum/1, Switch/3
  Memory/1 -> Switch/1
  Switch/1 -> Sum/2, Memory/1

== system Controller_Sim/Controller/Joystick Parser/xbox_mapping/Button Timer4 ==
  note: Button timer
      | Button needs to be pressed for 0.25 seconds to register
  In : Inport
  Clock : Clock
  Memory : Memory
  Sum : Sum  Inputs=|+-
  Switch : Switch  Criteria=u2 > Threshold
  Switch1 : Switch  Criteria=u2 > Threshold  Threshold=0.25
  off : Constant  Value=0
  on : Constant
  Out : Outport
  wires:
  off/1 -> Switch1/3
  Sum/1 -> Switch1/2
  Switch1/1 -> Out/1
  on/1 -> Switch1/1
  In/1 -> Switch/2
  Clock/1 -> Sum/1, Switch/3
  Memory/1 -> Switch/1
  Switch/1 -> Sum/2, Memory/1

== system Controller_Sim/Controller/Joystick Parser/xbox_mapping/Button Timer5 ==
  note: Button timer
      | Button needs to be pressed for 0.25 seconds to register
  In : Inport
  Clock : Clock
  Memory : Memory
  Sum : Sum  Inputs=|+-
  Switch : Switch  Criteria=u2 > Threshold
  Switch1 : Switch  Criteria=u2 > Threshold  Threshold=0.25
  off : Constant  Value=0
  on : Constant
  Out : Outport
  wires:
  off/1 -> Switch1/3
  Sum/1 -> Switch1/2
  Switch1/1 -> Out/1
  on/1 -> Switch1/1
  In/1 -> Switch/2
  Clock/1 -> Sum/1, Switch/3
  Memory/1 -> Switch/1
  Switch/1 -> Sum/2, Memory/1

== system Controller_Sim/Controller/Joystick Parser/xbox_mapping/Button Timer6 ==
  note: Button timer
      | Button needs to be pressed for 0.25 seconds to register
  In : Inport
  Clock : Clock
  Memory : Memory
  Sum : Sum  Inputs=|+-
  Switch : Switch  Criteria=u2 > Threshold
  Switch1 : Switch  Criteria=u2 > Threshold  Threshold=0.25
  off : Constant  Value=0
  on : Constant
  Out : Outport
  wires:
  off/1 -> Switch1/3
  Sum/1 -> Switch1/2
  Switch1/1 -> Out/1
  on/1 -> Switch1/1
  In/1 -> Switch/2
  Clock/1 -> Sum/1, Switch/3
  Memory/1 -> Switch/1
  Switch/1 -> Sum/2, Memory/1

== system Controller_Sim/Controller/Joystick Parser/xbox_mapping/Button Timer7 ==
  note: Button timer
      | Button needs to be pressed for 0.25 seconds to register
  In : Inport
  Clock : Clock
  Memory : Memory
  Sum : Sum  Inputs=|+-
  Switch : Switch  Criteria=u2 > Threshold
  Switch1 : Switch  Criteria=u2 > Threshold  Threshold=0.25
  off : Constant  Value=0
  on : Constant
  Out : Outport
  wires:
  off/1 -> Switch1/3
  Sum/1 -> Switch1/2
  Switch1/1 -> Out/1
  on/1 -> Switch1/1
  In/1 -> Switch/2
  Clock/1 -> Sum/1, Switch/3
  Memory/1 -> Switch/1
  Switch/1 -> Sum/2, Memory/1

== system Controller_Sim/Controller/Joystick Parser/xbox_mapping/Button Timer8 ==
  note: Button timer
      | Button needs to be pressed for 0.25 seconds to register
  In : Inport
  Clock : Clock
  Memory : Memory
  Sum : Sum  Inputs=|+-
  Switch : Switch  Criteria=u2 > Threshold
  Switch1 : Switch  Criteria=u2 > Threshold  Threshold=0.25
  off : Constant  Value=0
  on : Constant
  Out : Outport
  wires:
  off/1 -> Switch1/3
  Sum/1 -> Switch1/2
  Switch1/1 -> Out/1
  on/1 -> Switch1/1
  In/1 -> Switch/2
  Clock/1 -> Sum/1, Switch/3
  Memory/1 -> Switch/1
  Switch/1 -> Sum/2, Memory/1

== system Controller_Sim/Controller/Joystick Parser/xbox_mapping/Button Timer9 ==
  note: Button timer
      | Button needs to be pressed for 0.25 seconds to register
  In : Inport
  Clock : Clock
  Memory : Memory
  Sum : Sum  Inputs=|+-
  Switch : Switch  Criteria=u2 > Threshold
  Switch1 : Switch  Criteria=u2 > Threshold  Threshold=0.25
  off : Constant  Value=0
  on : Constant
  Out : Outport
  wires:
  off/1 -> Switch1/3
  Sum/1 -> Switch1/2
  Switch1/1 -> Out/1
  on/1 -> Switch1/1
  In/1 -> Switch/2
  Clock/1 -> Sum/1, Switch/3
  Memory/1 -> Switch/1
  Switch/1 -> Sum/2, Memory/1

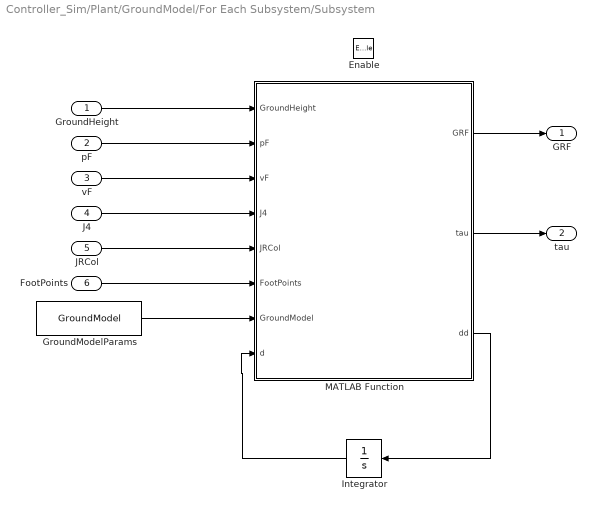
== system Controller_Sim/Plant/GroundModel/For Each Subsystem/Subsystem ==
  GroundHeight : Inport
  pF : Inport  Port=2
  vF : Inport  Port=3
  J4 : Inport  Port=4
  JRCol : Inport  Port=5
  FootPoints : Inport  Port=6
  Enable : EnablePort  StatesWhenEnabling=reset
  GroundModelParams : Constant  Value=GroundModel  OutDataTypeStr=Bus: GroundModelParamsBus
  Integrator : Integrator  InitialCondition=[0; 0]
  MATLAB Function : MATLAB Function  TreatAsAtomicUnit=on
  GRF : Outport  OutputWhenDisabled=reset  InitialOutput=[0;0;0]
  tau : Outport  Port=2  OutputWhenDisabled=reset  InitialOutput=zeros(16,1)
  wires:
  GroundModelParams/1 -> MATLAB Function/7(GroundModel)
  MATLAB Function/3(dd) -> Integrator/1
  Integrator/1 -> MATLAB Function/8(d)
  vF/1 -> MATLAB Function/3(vF)
  pF/1 -> MATLAB Function/2(pF)
  MATLAB Function/1(GRF) -> GRF/1
  MATLAB Function/2(tau) -> tau/1
  J4/1 -> MATLAB Function/4(J4)
  JRCol/1 -> MATLAB Function/5(JRCol)
  FootPoints/1 -> MATLAB Function/6(FootPoints)
  GroundHeight/1 -> MATLAB Function/1(GroundHeight)

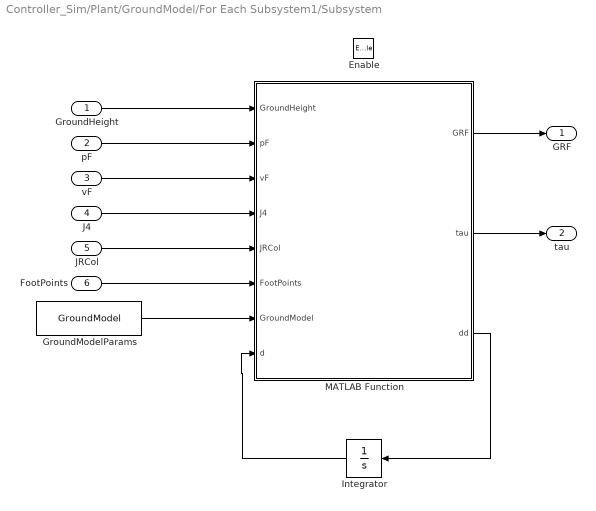
== system Controller_Sim/Plant/GroundModel/For Each Subsystem1/Subsystem ==
  GroundHeight : Inport
  pF : Inport  Port=2
  vF : Inport  Port=3
  J4 : Inport  Port=4
  JRCol : Inport  Port=5
  FootPoints : Inport  Port=6
  Enable : EnablePort  StatesWhenEnabling=reset
  GroundModelParams : Constant  Value=GroundModel  OutDataTypeStr=Bus: GroundModelParamsBus
  Integrator : Integrator  InitialCondition=[0; 0]
  MATLAB Function : MATLAB Function  TreatAsAtomicUnit=on
  GRF : Outport  OutputWhenDisabled=reset  InitialOutput=[0;0;0]
  tau : Outport  Port=2  OutputWhenDisabled=reset  InitialOutput=zeros(16,1)
  wires:
  GroundHeight/1 -> MATLAB Function/1(GroundHeight)
  FootPoints/1 -> MATLAB Function/6(FootPoints)
  JRCol/1 -> MATLAB Function/5(JRCol)
  J4/1 -> MATLAB Function/4(J4)
  MATLAB Function/2(tau) -> tau/1
  MATLAB Function/1(GRF) -> GRF/1
  pF/1 -> MATLAB Function/2(pF)
  vF/1 -> MATLAB Function/3(vF)
  Integrator/1 -> MATLAB Function/8(d)
  MATLAB Function/3(dd) -> Integrator/1
  GroundModelParams/1 -> MATLAB Function/7(GroundModel)

== matlab function Controller_Sim/Plant/GroundModel/For Each Subsystem1/Subsystem/MATLAB Function ==
  data: GroundHeight input; pF input; GRF output; tau output; vF input; J4 input; JRCol input; FootPoints input; GroundModel input; d input; dd output
function [GRF, tau, dd] = computeLuGreHertzian(GroundHeight, pF, vF, J4, JRCol, FootPoints, GroundModel, d)
    %#codegen
    
    [F, dd] = LuGreHertzian(pF(3), vF(3,:), d, vF(1:2,:), GroundModel,GroundHeight);
    GRF = F(:);
    
    J   = J4 + FootPoints(1)*JRCol(1:3,:) + FootPoints(2)*JRCol(4:6,:) + FootPoints(3)*JRCol(7:9,:);
    tau = J.'*GRF;
end

== matlab function Controller_Sim/Plant/Robot/Dynamics ==
  data: x input; u input; D input; Cdq input; G input; B input; FGround input; Fstiction input; x_dot output; spring_k parameter; spring_zeta parameter; ExternalHipForce input; Ttime input
function x_dot  = ATRIAS3D_Flight(x, u, D, Cdq, G, B, FGround, Fstiction, spring_k, spring_zeta, ExternalHipForce,Ttime)
%#codegen

q  = x(1:16);
dq = x(17:32);

% Lagrange model
%[D,Cdq,G,B,J_yaw,dJ_yaw] = ATRIAS3D_Lagrange_Hip(q,dq);

%Calculate spring and damper forces
[K_spring, K_damping] = ATRIAS3D_Spring_Constants(spring_k, spring_zeta);
FSpring = K_spring * q + K_damping * dq; 

% Calculate the H vector
H = Cdq + G + FSpring - FGround - B*(u - Fstiction);

% PUSH START
% H(1) = H(1) + 0.5*ExternalHipForce;
% if Ttime < 10
%     H(2) = H(2) + 1*ExternalHipForce;
% else
%     H(2) = H(2) + 0*ExternalHipForce;
% end

kpboom = 10000;
kdboom = 1000;

H(4) = H(4)+kdboom/10*dq(4);  % Yaw friction constraint

%  ---------- TESTS ------------------
isTest_holdInAir = true;
isTest_doubleSupport = false;
isTest_constantHip = false;


if isTest_holdInAir
	H(1) = H(1)+kpboom*(q(1))+kdboom*dq(1);   % Side
	H(2) = H(2)+kpboom*(q(2))+kdboom*dq(2);   % Side
	H(3) = H(3)+kpboom*(q(3)-1.5)+kdboom*dq(3); % Hang in the air
	H(4:5) = H(4:5)+kpboom*(q(4:5)-[0*pi/180;0*pi/180])+kdboom*dq(4:5);   % Yaw and Roll
	H(6) = H(6)+kpboom*(q(6)-0*pi/180)+kdboom*dq(6);
end

if isTest_doubleSupport
	if (Ttime < 3)
		H(6) = H(6)+kpboom*(q(6)-0*pi/180)+kdboom*dq(6);
		H(3) = H(3)+kpboom*(q(3)-1.1)+kdboom*dq(3); % Hang in the air
		H(4:5) = H(4:5)+kpboom*(q(4:5)-[0;0])+kdboom*dq(4:5);   % Yaw and Roll
	end
	H(1) = H(1)+kpboom*(q(1))+kdboom*dq(1);   % Side
	H(2) = H(2)+kpboom*(q(2))+kdboom*dq(2);   % Side
end

if isTest_constantHip
	H(1) = H(1)+kpboom*(q(1))+kdboom*dq(1);   % Side
	H(2) = H(2)+kpboom*(q(2))+kdboom*dq(2);   % Side
end

%  ------------------------------------

	
if 0
%     H(1) = H(1)+kpboom*(q(1))+kdboom*dq(1);   % Side
%     H(4:5) = H(4:5)+kpboom*(q(4:5)-[0;0])+kdboom*dq(4:5);   % Yaw and Roll
%     H(4) = H(4)+kpboom*(q(4)-[0])+kdboom*dq(4);   % Yaw
% 	if dq(4)>0
		H(4) = H(4)+kdboom/100*dq(4);   % Yaw
% 	else
% 		H(4) = H(4)+kdboom/10*dq(4);   % Yaw
% 	end
%     if Ttime < 1
    if (Ttime < 0) || (Ttime < 0)
        H([6]) = H([6])+kpboom*(q([6])-[0*pi/180])+kdboom*dq([6]); 
%         if Ttime < 1
%           % Pitch
          
%         H([2,3]) = H([2,3])+kpboom*(q([2,3])-[0;1.1])+kdboom*dq([2,3]); % Hang in the air
        H(3) = H(3)+kpboom*(q(3)-1.1)+kdboom*dq(3); % Hang in the air

%         else
%         H([2]) = H([2])+kpboom*(q([2])-[0])+kdboom*dq([2]);       % Hold in  place
%         end
%     H(1) = H(1)+kpboom*(q(1))+kdboom*dq(1);   % Side
%     H(4:5) = H(4:5)+kpboom*(q(4:5)-[0;-0])+kdboom*dq(4:5);   % Roll and Yaw

        H(1) = H(1)+kpboom*(q(1))+kdboom*dq(1);   % Side
        H(4:5) = H(4:5)+kpboom*(q(4:5)-[0;0])+kdboom*dq(4:5);   % Yaw and Roll
    end
end
% D = D + 0.1*rand(size(D));
% H = H + 0.2*rand(size(H));

ddq = -D\H;
x_dot = [dq;ddq];

%--------------------------------------------------------------------------

== matlab function Controller_Sim/Plant/GroundModel/For Each Subsystem/Subsystem/MATLAB Function ==
  data: GroundHeight input; pF input; GRF output; tau output; vF input; J4 input; JRCol input; FootPoints input; GroundModel input; d input; dd output
function [GRF, tau, dd] = computeLuGreHertzian(GroundHeight, pF, vF, J4, JRCol, FootPoints, GroundModel, d)
    %#codegen
    
    [F, dd] = LuGreHertzian(pF(3), vF(3,:), d, vF(1:2,:), GroundModel,GroundHeight);
    GRF = F(:);
    
    J   = J4 + FootPoints(1)*JRCol(1:3,:) + FootPoints(2)*JRCol(4:6,:) + FootPoints(3)*JRCol(7:9,:);
    tau = J.'*GRF;
end

== matlab function Controller_Sim/Plant/extract ==
  data: x input; q output; dq output
function [q,dq] = extract(x)
%#codegen
q = x(1:16,1);
dq = x(17:32,1);

== matlab function Controller_Sim/Plant/Robot/MATLAB Function ==
  data: q input; D output; dq input; leg_length input; Cdq output; G output; B output; torso_com_offset input
function [D, Cdq, G, B] = Compute_Lagrange_Model(q, dq, leg_length, torso_com_offset)
%#codegen

% Call functions generated from symbolic model
extra_vars = [leg_length; torso_com_offset];
D = OriginalLeg_Springs_VariableLeg_COMoffset.ATRIAS3D_D_Hip(q,extra_vars);
Cdq = OriginalLeg_Springs_VariableLeg_COMoffset.ATRIAS3D_Cdq_Hip(q,dq,extra_vars);
G = OriginalLeg_Springs_VariableLeg_COMoffset.ATRIAS3D_G_Hip(q,extra_vars);
B = OriginalLeg_Springs_VariableLeg_COMoffset.ATRIAS3D_B_Hip(q);

== matlab function Controller_Sim/Controller/MATLAB Function ==
  data: u_new input; u_old output
function u_old = Convert_u_to_old_coordinates(u_new)
%#codegen

% u_new = [qHR, qAR, qBR, qHL, qAL, qBL]
% u_old = [qAR, qBR, qHR, qAL, qBL, qHL]

u_old = u_new([2,3,1,5,6,4]);
u_old(6) = -u_old(6); % Flip left hip torque

end

== matlab function Controller_Sim/Controller/MATLAB Function1 ==
  data: q_old input; q_new output; dq_old input; dq_new output
function [q_new, dq_new] = Convert_x_to_new_coordinates(q_old, dq_old)
%#codegen
q_new = zeros(17,1);
dq_new = zeros(17,1);

% q_new = [pitch; roll; yaw;
%          qHR; qAR; qBR; qAgrR; qBgrR; FourBarAR; FourBarBR;
%          qHL; qAL; qBL; qAgrL; qBgrL; FourBarAL; FourBarBL];

% Orientation
q_new(1:3,:) = q_old([3,2,1],:); 
dq_new(1:3,:) = dq_old([3,2,1],:); 

% Right Side
q_new(4:8,:) = q_old([10,4,5,8,9],:); 
dq_new(4:8,:) = dq_old([10,4,5,8,9],:); 
q_new(9:10,:) = q_old([5,4]) - q_old([4,5]);
dq_new(9:10,:) = dq_old([5,4]) - dq_old([4,5]);


% Left Side
q_new(11:15,:) = q_old([13,6,7,11,12],:); 
dq_new(11:15,:) = dq_old([13,6,7,11,12],:); 
q_new(16:17,:) = q_old([7,6]) - q_old([6,7]);
dq_new(16:17,:) = dq_old([7,6]) - dq_old([6,7]);
q_new(11) = -q_new(11);
dq_new(11) = -dq_new(11);


end

== matlab function Controller_Sim/Subsystem/MATLAB Function ==
  data: q input; leg_length input; torso_com_offset input
function Animation(q, leg_length, torso_com_offset)
%#codegen 
persistent f p1HR p2HR p31R p42R pHR0TR p1HL p2HL p31L p42L pHR0TL torso
leg1Color = 'r'; 
leg2Color = 'b';
torsoColor = 'k';
groundColor = 'g';
        
% Get Positions
[pcm, p0, p0T, pHR, p1R, p2R, p3R, p4R, pHL, p1L, p2L, p3L, p4L] =  OriginalLeg_Springs_VariableLeg_COMoffset.ATRIAS3D_Positions_Hip(q,[leg_length;torso_com_offset]);

if isempty(f)
    f = figure;
    
    % Define stance leg
    p1HR = line([p1R(1) pHR(1)],[p1R(2) pHR(2)],[p1R(3) pHR(3)]);
    p2HR = line([p2R(1) pHR(1)],[p2R(2) pHR(2)],[p2R(3) pHR(3)]);
    p31R = line([p3R(1) p1R(1)],[p3R(2) p1R(2)],[p3R(3) p1R(3)]);
    p42R = line([p4R(1) p2R(1)],[p4R(2) p2R(2)],[p4R(3) p2R(3)]);
    pHR0TR = line([p0(1) pHR(1)],[p0(2) pHR(2)],[p0(3) pHR(3)]);
    
    set(p1HR,'LineWidth',3,'Color',leg1Color);
    set(p2HR,'LineWidth',3,'Color',leg1Color);
    set(p31R,'LineWidth',3,'Color',leg1Color);
    set(p42R,'LineWidth',3,'Color',leg1Color);
    set(pHR0TR,'LineWidth',3,'Color',torsoColor);
    
    % Define swing leg
    p1HL = line([p1L(1) pHL(1)],[p1L(2) pHL(2)],[p1L(3) pHL(3)]);
    p2HL = line([p2L(1) pHL(1)],[p2L(2) pHL(2)],[p2L(3) pHL(3)]);
    p31L = line([p3L(1) p1L(1)],[p3L(2) p1L(2)],[p3L(3) p1L(3)]);
    p42L = line([p4L(1) p2L(1)],[p4L(2) p2L(2)],[p4L(3) p2L(3)]);
    pHR0TL = line([p0(1) pHL(1)],[p0(2) pHL(2)],[p0(3) pHL(3)]);
    
    set(p1HL,'LineWidth',3,'Color',leg2Color);
    set(p2HL,'LineWidth',3,'Color',leg2Color);
    set(p31L,'LineWidth',3,'Color',leg2Color);
    set(p42L,'LineWidth',3,'Color',leg2Color);
    set(pHR0TL,'LineWidth',3,'Color',torsoColor);
    
    % Define torso
    torso = line([p0(1) p0T(1)], [p0(2) p0T(2)], [p0(3) p0T(3)]);
    set(torso,'LineWidth',3,'Color',torsoColor);

end

figure(f);
axis([pcm(1)-1, pcm(1)+1, pcm(2)-1, pcm(2)+1, 0 2 0 1]);

set(p1HR,'XData',[p1R(1) pHR(1)],'YData',[p1R(2) pHR(2)],'ZData',[p1R(3) pHR(3)]);
set(p2HR,'XData',[p2R(1) pHR(1)],'YData',[p2R(2) pHR(2)],'ZData',[p2R(3) pHR(3)]);
set(p31R,'XData',[p3R(1) p1R(1)],'YData',[p3R(2) p1R(2)],'ZData',[p3R(3) p1R(3)]);
set(p42R,'XData',[p4R(1) p2R(1)],'YData',[p4R(2) p2R(2)],'ZData',[p4R(3) p2R(3)]);
set(pHR0TR,'XData',[p0(1) pHR(1)],'YData',[p0(2) pHR(2)],'ZData',[p0(3) pHR(3)]);

set(p1HL,'XData',[p1L(1) pHL(1)],'YData',[p1L(2) pHL(2)],'ZData',[p1L(3) pHL(3)]);
set(p2HL,'XData',[p2L(1) pHL(1)],'YData',[p2L(2) pHL(2)],'ZData',[p2L(3) pHL(3)]);
set(p31L,'XData',[p3L(1) p1L(1)],'YData',[p3L(2) p1L(2)],'ZData',[p3L(3) p1L(3)]);
set(p42L,'XData',[p4L(1) p2L(1)],'YData',[p4L(2) p2L(2)],'ZData',[p4L(3) p2L(3)]);
set(pHR0TL,'XData',[p0(1) pHL(1)],'YData',[p0(2) pHL(2)],'ZData',[p0(3) pHL(3)]);

set(torso,'XData',[p0(1) p0T(1)],'YData',[p0(2) p0T(2)],'ZData',[p0(3) p0T(3)]);

== matlab function Controller_Sim/Plant/GroundModel/MATLAB Function ==
  data: x input; pR output; vR output; J4R output; JR1Col output; pL output; vL output; J4L output; JR5Col output; FootPoints input; leg_length input; torso_com_offset input
function [pR, vR, J4R, JR1Col, pL, vL, J4L, JR5Col] = getFootHeightAndVelocity(x, FootPoints,  leg_length, torso_com_offset)
    %#codegen
    [pR, vR, J4R, JR1Col, pL, vL, J4L, JR5Col] = FootHeightAndVelocity(x, FootPoints, leg_length, torso_com_offset);
end
